simulink model "Exercitiul1"  (R2016a)
settings: Solver=VariableStepDiscrete  StartTime=0.0  StopTime=100  RelTol=1e-3
undefined symbols (not defined in the file): m, n
settings Model: Creator=Cristina  LastModifiedBy=Cristina

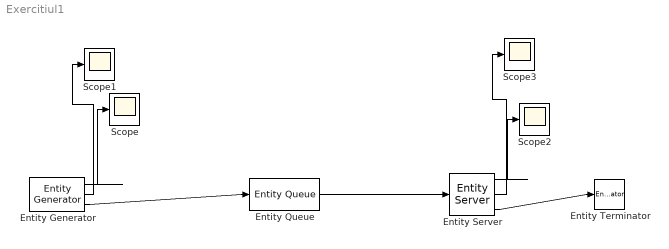
== system Exercitiul1 ==
  Entity Generator : EntityGenerator  OutputPortMessageModes=n,n,m  TimeSource=MATLAB action  IntergenerationTimeAction=dt = 0.8 * rand + 0.2  NumberEntitiesDeparted=on  AverageIntergenerationTime=on  EntityType=Structured  EntityTypeName=Entity
      settings: OutputPortMap=o0,o2,o3
  Entity Queue : EntityQueue  InputPortMessageModes=m  OutputPortMessageModes=m  Capacity=inf
      settings: OutputPortMap=o5
  Entity Server : EntityServer  InputPortMessageModes=m  OutputPortMessageModes=n,n,m  Capacity=1  ServiceTimeSource=MATLAB action  ServiceTimeAction=dt = 0.3 + 0.9 * rand;  NumberEntitiesDeparted=on  AverageWait=on
      settings: OutputPortMap=o0,o4,o9
  Entity Terminator : EntityTerminator  InputPortMessageModes=m
  Scope{,1..3} (4 alike) : Scope
  wires:
  Entity Server/3 -> Entity Terminator/1
  Entity Queue/1 -> Entity Server/1
  Entity Generator/3 -> Entity Queue/1
  Entity Generator/1 -> Scope/1
  Entity Generator/2 -> Scope1/1
  Entity Server/1 -> Scope2/1
  Entity Server/2 -> Scope3/1
